simulink model "Pendulo"  (R2021a)
settings: Solver=VariableStepAuto  StartTime=0.0  StopTime=30  RelTol=1e-3
settings Model: Creator=benja  LastModifiedBy=benja

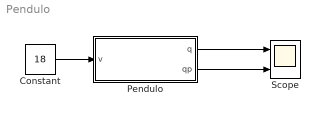
== system Pendulo ==
  Constant : Constant  Value=18
  Pendulo : Subsystem
  Scope : Scope  NumInputPorts=2
  wires:
  Constant/1 -> Pendulo/1(v)
  Pendulo/1(q) -> Scope/1
  Pendulo/2(qp) -> Scope/2

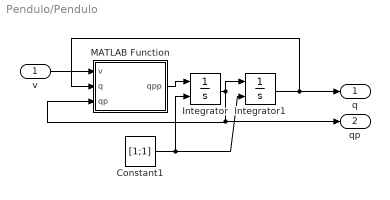
== system Pendulo/Pendulo ==
  v : Inport
  Constant1 : Constant  Value=[1;1]
  Integrator : Integrator  InitialConditionSource=external
  Integrator1 : Integrator  InitialConditionSource=external
  MATLAB Function : MATLAB Function  TreatAsAtomicUnit=on
  q : Outport
  qp : Outport  Port=2
  wires:
  Integrator/1 -> Integrator1/1, qp/1, MATLAB Function/3(qp)
  Constant1/1 -> Integrator1/2, Integrator/2
  v/1 -> MATLAB Function/1(v)
  Integrator1/1 -> q/1, MATLAB Function/2(q)
  MATLAB Function/1(qpp) -> Integrator/1

== matlab function Pendulo/MATLAB Function ==
  data: v input; qpp output; q input; qp input
function qpp  = fcn(v,q,qp)
m = 1
l = 1
g = 9.81
mb = 1
lb = 1
r = 1;
fm = 1
fL = 1
Ka = 1;
Kb = 1;
Ra = 1;

Jm1 = 1;
Jm2 = 1;
Jm = [Jm1 0; 0 Jm2]
J = [Jm1 0;0 Jm2]

JL = J + m*l^2
KL = (mb*lb+m*l)*g

qpp = inv(Jm+JL/r^2)*((Ka/(r*Ra))*v-(KL/r^2)*sin(q)-(fm+(fL/r^2)+(Ka*Kb)/(r*Ra))*qp)
